simulink model "unittest_PX4SITLSFunc"  (R2024a)
settings: Solver=VariableStepAuto  StartTime=0.0  StopTime=10.0  RelTol=1e-3
libraries: SignalEditorBlockLib x1, library_PX4SITLSFunc x1
settings Model: Creator=tommy  LastModifiedBy=tommy

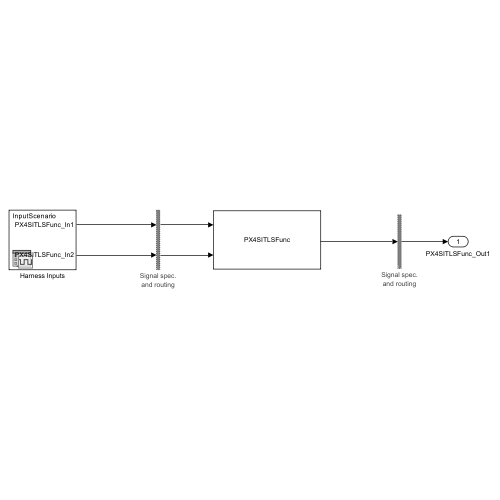
[thumbnail: Simulink's stored preview of the top-level diagram]
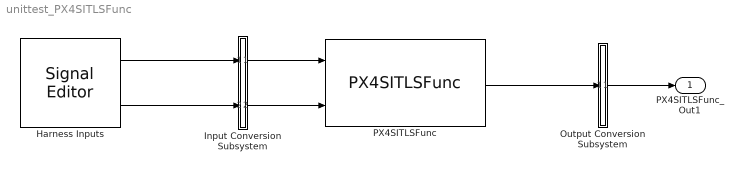
== system unittest_PX4SITLSFunc ==
  Harness Inputs : SignalEditorBlockLib/Signal Editor  FileName=harness_PX4SITLSFunc_HarnessInputs.mat  ActiveScenario=InputScenario  ActiveSignal=PX4SITLSFunc_In2  IsBus=off  OutputBusObjectStr=Bus: BusObject  SampleTime=[0, 1]  Interpolate=off  ZeroCross=off  OutputAfterFinalValue=Setting to zero  Unit=inherit  PreserveSignalName=on  ApplySigPropsToAllScenarios=on  ApplySigPropsToAllSignals=off
  Input Conversion Subsystem : Subsystem  Tag=__SLT_ICS__  Description=|
      | Signal spec.
      | and routing
      settings: AttributesFormatString=%<Description>
  Output Conversion Subsystem : Subsystem  Tag=__SLT_OCS__  Description=|
      | Signal spec.
      | and routing
      settings: AttributesFormatString=%<Description>
  PX4SITLSFunc : library_PX4SITLSFunc/PX4SITLSFunc
  PX4SITLSFunc_Out1 : Outport
  wires:
  Harness Inputs/1 -> Input Conversion Subsystem/1(Inport_1)
  Harness Inputs/2 -> Input Conversion Subsystem/2(Inport_2)
  Output Conversion Subsystem/1(Outport_1) -> PX4SITLSFunc_Out1/1
  Input Conversion Subsystem/1(Outport_1) -> PX4SITLSFunc/1
  Input Conversion Subsystem/2(Outport_2) -> PX4SITLSFunc/2
  PX4SITLSFunc/1 -> Output Conversion Subsystem/1(Inport_1)

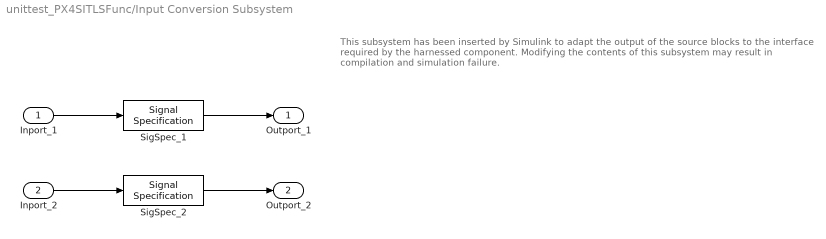
== system unittest_PX4SITLSFunc/Input Conversion Subsystem ==
  note: This subsystem has been inserted by Simulink to adapt the output of the source blocks to the interface required by the harnessed component.
      |  Modifying the contents of this subsystem may result in compilation and simulation failure.
  Inport_1 : Inport
  Inport_2 : Inport  Port=2
  SigSpec_1 : SignalSpecification  OutDataTypeStr=double  Dimensions=[1024]  SampleTime=[0, 1]
  SigSpec_2 : SignalSpecification  OutDataTypeStr=double  Dimensions=[1024]  SampleTime=[0, 1]
  Outport_1 : Outport
  Outport_2 : Outport  Port=2
  wires:
  SigSpec_1/1 -> Outport_1/1
  Inport_1/1 -> SigSpec_1/1
  SigSpec_2/1 -> Outport_2/1
  Inport_2/1 -> SigSpec_2/1

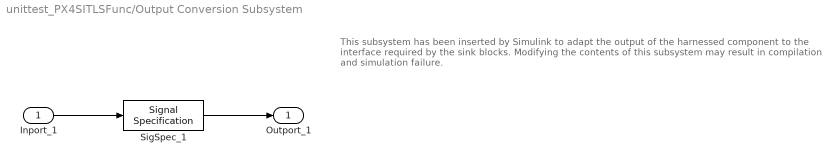
== system unittest_PX4SITLSFunc/Output Conversion Subsystem ==
  note: This subsystem has been inserted by Simulink to adapt the output of the harnessed component to the interface required by the sink blocks.
      |  Modifying the contents of this subsystem may result in compilation and simulation failure.
  Inport_1 : Inport
  SigSpec_1 : SignalSpecification  OutDataTypeStr=double  Dimensions=[16]
  Outport_1 : Outport
  wires:
  Inport_1/1 -> SigSpec_1/1
  SigSpec_1/1 -> Outport_1/1
